simulink model "plant_n"  (R2023a)
settings: Solver=FixedStepAuto  StartTime=0.0  StopTime=200  FixedStep=0.01  RelTol=1e-3
values from neighbouring files (symbols this model uses):
  filter_3 = conv([0.1,1],conv([0.1 1],[0.1 1]))    [main_proj.m]
  filter_x = conv([0.7,1],conv([0.7 1],[0.7 1]))    [main_proj.m]
  kd = 1.117    [main_proj.m]
  ki = 4.47    [main_proj.m]
  kp = 5.366    [main_proj.m]
libraries: neural x772, slpidlib x6
(part 20 of 26)

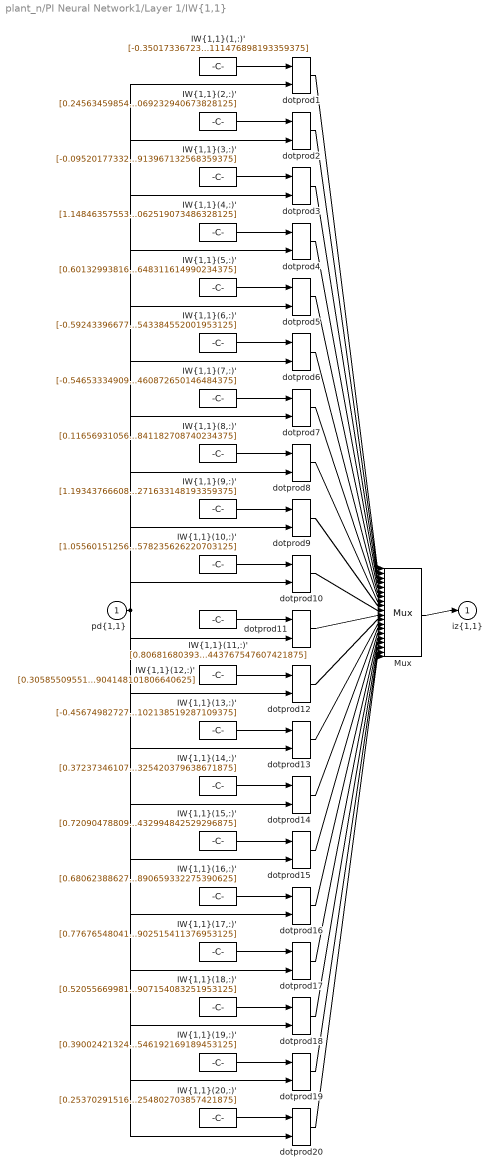
== system plant_n/PI Neural Network1/Layer 1/IW{1,1} ==
  "pd{1,1}" : Inport  PortDimensions=12  SampleTime=0.01
      mask Display: e = 0.06;c1 = [120 230 180]/255;c2 = ([120 230 180]+0)/(256+128);c3 = ([120 230 180]+128)/(256+128);patch([0 1 1 0],[0 0 1 1],c1);patch([0 1 1 1-e 1-e 0+e],[0 0 1 1-e 0+e 0+e],c2);patch([0 0 1 1-e 0+e 0+e],[0 1 1 1-e 1-e 0+e],c3);plot([0 1 1 0 0],[0 0 1 1 0]);
  "IW{1,1}(1,:)'" : Constant  Value=[-0.3501733672305566980043067815131507813930511474609375;0.21065488893706219020174330580630339682102203369140625;-0.210989136698746027054340856921044178307056427001953125;-0.33078704563438676711228936255793087184429168701171875;0.62945158155652103371124894692911766469478607177734375;0.5671066900211059191860840655863285064697265625;0.7803009476457349880007541287341155111789703369140625;-0.168810783126756736027829219892737455666065216064453125;0.980768973519757114587491741986013948917388916015625;-0.84484218705403490989880310735316015779972076416015625;-0.0895432947846148963311208035520394332706928253173828125;-0.9561220185730545662039503440610133111476898193359375]
      mask Display: e = 0.06;c1 = [120 150 230]/255;c2 = ([120 150 230]+0)/383;c3 = ([120 150 230]+128)/383;patch([0 1 1 0],[0 0 1 1],c1);patch([0 1 1 1-e 1-e 0+e],[0 0 1 1-e 0+e 0+e],c2);patch([0 0 1 1-e 0+e 0+e],[0 1 1 1-e 1-e 0+e],c3);plot([0 1 1 0 0],[0 0 1 1 0]);disp('Weights');
  "IW{1,1}(10,:)'" : Constant  Value=[1.05560151256634693339719888172112405300140380859375;0.9332939344408643922434976047952659428119659423828125;-0.277691460157354408355701025357120670378208160400390625;0.7060845075612072196946655822102911770343780517578125;-0.09695879864153743310506428088046959601342678070068359375;-0.2443508749205889341027386763016693294048309326171875;0.367614281091130312706383165277657099068164825439453125;-0.454827087842074317958207529954961501061916351318359375;-0.1513157236805418859315608415272436104714870452880859375;-0.59870946189401774706340120246750302612781524658203125;0.58984455881189068460201951893395744264125823974609375;-0.27134154152465239651093042994034476578235626220703125]
      mask Display: e = 0.06;c1 = [120 150 230]/255;c2 = ([120 150 230]+0)/383;c3 = ([120 150 230]+128)/383;patch([0 1 1 0],[0 0 1 1],c1);patch([0 1 1 1-e 1-e 0+e],[0 0 1 1-e 0+e 0+e],c2);patch([0 0 1 1-e 0+e 0+e],[0 1 1 1-e 1-e 0+e],c3);plot([0 1 1 0 0],[0 0 1 1 0]);disp('Weights');
  "IW{1,1}(11,:)'" : Constant  Value=[0.80681680393463273137655278333113528788089752197265625;0.09439694486195693290397912278422154486179351806640625;-0.77701084247417007144775880078668706119060516357421875;-0.427850899211101032282300593578838743269443511962890625;-0.2232987875497577656691561287516378797590732574462890625;-0.803257944648623212202664944925345480442047119140625;-0.5029394327736536052242399819078855216503143310546875;0.51929065478912439512981791267520748078823089599609375;-0.337093294264546095018175719815189950168132781982421875;-0.834341251775934100720633068704046308994293212890625;0.9091864342576430058073810869245789945125579833984375;-0.89888560861707400562181646819226443767547607421875]
      mask Display: e = 0.06;c1 = [120 150 230]/255;c2 = ([120 150 230]+0)/383;c3 = ([120 150 230]+128)/383;patch([0 1 1 0],[0 0 1 1],c1);patch([0 1 1 1-e 1-e 0+e],[0 0 1 1-e 0+e 0+e],c2);patch([0 0 1 1-e 0+e 0+e],[0 1 1 1-e 1-e 0+e],c3);plot([0 1 1 0 0],[0 0 1 1 0]);disp('Weights');
  "IW{1,1}(12,:)'" : Constant  Value=[0.305855095510365881938952270502340979874134063720703125;0.1233616864154553904864286550946417264640331268310546875;-0.56671614694551519786358539931825362145900726318359375;-0.56492851509072072868633540565497241914272308349609375;0.1722457842120801718710509931042906828224658966064453125;0.63864705288493739399058313210844062268733978271484375;-0.943134606258703822589950505062006413936614990234375;0.80407771540784123143197348326793871819972991943359375;-0.256012471713641887038903632856090553104877471923828125;0.77675127860351655950665872296667657792568206787109375;-0.86701208832907961099323301823460496962070465087890625;0.85618857861038721868141010418185032904148101806640625]
      mask Display: e = 0.06;c1 = [120 150 230]/255;c2 = ([120 150 230]+0)/383;c3 = ([120 150 230]+128)/383;patch([0 1 1 0],[0 0 1 1],c1);patch([0 1 1 1-e 1-e 0+e],[0 0 1 1-e 0+e 0+e],c2);patch([0 0 1 1-e 0+e 0+e],[0 1 1 1-e 1-e 0+e],c3);plot([0 1 1 0 0],[0 0 1 1 0]);disp('Weights');
  "IW{1,1}(13,:)'" : Constant  Value=[-0.456749827277473485764858196489512920379638671875;-0.70461220297198046136344373735482804477214813232421875;-0.209279497403218883722075815967400558292865753173828125;0.41399815885431345829914562273188494145870208740234375;0.89381430939822548165096804950735531747341156005859375;0.84335366269535050331995762462611310184001922607421875;0.0676310309392321451493756967465742491185665130615234375;-0.57820143903720777611709991106181405484676361083984375;0.0861819469902399826199967947104596532881259918212890625;-0.01237860880424513677910969278173070051707327365875244140625;-0.660821274311004902557442619581706821918487548828125;0.35180784796509489975591122856712900102138519287109375]
      mask Display: e = 0.06;c1 = [120 150 230]/255;c2 = ([120 150 230]+0)/383;c3 = ([120 150 230]+128)/383;patch([0 1 1 0],[0 0 1 1],c1);patch([0 1 1 1-e 1-e 0+e],[0 0 1 1-e 0+e 0+e],c2);patch([0 0 1 1-e 0+e 0+e],[0 1 1 1-e 1-e 0+e],c3);plot([0 1 1 0 0],[0 0 1 1 0]);disp('Weights');
  "IW{1,1}(14,:)'" : Constant  Value=[0.372373461077679379638283307940582744777202606201171875;-0.38560447648762530281629778983187861740589141845703125;0.34196789986070263989148543259943835437297821044921875;-0.50526431518178716029154884381568990647792816162109375;-0.167743758165300960172316990792751312255859375;0.84873249279830620395159712643362581729888916015625;-0.94999636271671772380642551070195622742176055908203125;0.860639973471389652104335254989564418792724609375;0.7117112004407477598988407407887279987335205078125;0.97995227919054084253502878709696233272552490234375;-0.4320334908905001380929888910031877458095550537109375;-0.9055841713231955747431811687420122325420379638671875]
      mask Display: e = 0.06;c1 = [120 150 230]/255;c2 = ([120 150 230]+0)/383;c3 = ([120 150 230]+128)/383;patch([0 1 1 0],[0 0 1 1],c1);patch([0 1 1 1-e 1-e 0+e],[0 0 1 1-e 0+e 0+e],c2);patch([0 0 1 1-e 0+e 0+e],[0 1 1 1-e 1-e 0+e],c3);plot([0 1 1 0 0],[0 0 1 1 0]);disp('Weights');
  "IW{1,1}(15,:)'" : Constant  Value=[0.72090478809743185895086980963242240250110626220703125;-0.964711239579766566265561777981929481029510498046875;-0.269719016390192634080591460588038899004459381103515625;-0.245333648835221740380774235745775513350963592529296875;-0.5506486579344376242062253368203528225421905517578125;-0.73357525751399033087096768213086761534214019775390625;0.58313879853820960175170284855994395911693572998046875;0.79142205377866881033099843989475630223751068115234375;0.160230341602728809657918418452027253806591033935546875;0.584078718962899756661499850451946258544921875;0.485155412787328932378017043447471223771572113037109375;0.65783015821145607304742952692322432994842529296875]
      mask Display: e = 0.06;c1 = [120 150 230]/255;c2 = ([120 150 230]+0)/383;c3 = ([120 150 230]+128)/383;patch([0 1 1 0],[0 0 1 1],c1);patch([0 1 1 1-e 1-e 0+e],[0 0 1 1-e 0+e 0+e],c2);patch([0 0 1 1-e 0+e 0+e],[0 1 1 1-e 1-e 0+e],c3);plot([0 1 1 0 0],[0 0 1 1 0]);disp('Weights');
  "IW{1,1}(16,:)'" : Constant  Value=[0.6806238862716977866540446484577842056751251220703125;0.30321005464548689278814208591938950121402740478515625;-0.397392951058915755435663186290184967219829559326171875;-0.372547888856498865539634834931348450481891632080078125;0.1705807666146650081184787950405734591186046600341796875;0.61134879168408728933314932874054647982120513916015625;0.715307662324553117372261112905107438564300537109375;-0.6937658001944537744520857813768088817596435546875;-0.1384741823775422486786368381217471323907375335693359375;-0.5544804190145942168754800150054506957530975341796875;-0.77165132177390471923672521370463073253631591796875;-0.95013052194457225940737998826080001890659332275390625]
      mask Display: e = 0.06;c1 = [120 150 230]/255;c2 = ([120 150 230]+0)/383;c3 = ([120 150 230]+128)/383;patch([0 1 1 0],[0 0 1 1],c1);patch([0 1 1 1-e 1-e 0+e],[0 0 1 1-e 0+e 0+e],c2);patch([0 0 1 1-e 0+e 0+e],[0 1 1 1-e 1-e 0+e],c3);plot([0 1 1 0 0],[0 0 1 1 0]);disp('Weights');
  "IW{1,1}(17,:)'" : Constant  Value=[0.77676548041798110233457919093780219554901123046875;0.59875298284257361114413242830778472125530242919921875;-0.6769123517311761428771887949551455676555633544921875;-0.33193049430556997858587919836281798779964447021484375;-0.818157794952087069617618908523581922054290771484375;-0.488999925412603453356297222853754647076129913330078125;-0.00514354018054317962960197974098264239728450775146484375;0.154838187918311442903274155469262041151523590087890625;-0.1370417754103717411506835333057097159326076507568359375;-0.0833729676382103102039167197290225885808467864990234375;0.2300759161553746212636184509392478503286838531494140625;0.1954796096302804375710593376425094902515411376953125]
      mask Display: e = 0.06;c1 = [120 150 230]/255;c2 = ([120 150 230]+0)/383;c3 = ([120 150 230]+128)/383;patch([0 1 1 0],[0 0 1 1],c1);patch([0 1 1 1-e 1-e 0+e],[0 0 1 1-e 0+e 0+e],c2);patch([0 0 1 1-e 0+e 0+e],[0 1 1 1-e 1-e 0+e],c3);plot([0 1 1 0 0],[0 0 1 1 0]);disp('Weights');
  "IW{1,1}(18,:)'" : Constant  Value=[0.5205566998138924095229640442994423210620880126953125;0.57546124158919287339131187763996422290802001953125;-0.61229287881037508523007772964774630963802337646484375;0.8385272354770882952124111398006789386272430419921875;-0.5968790319572521152480248929350636899471282958984375;-0.6583580586300550319123203735216520726680755615234375;0.77313243054862790248904502732330001890659332275390625;1.03942917397456557893065109965391457080841064453125;-0.4563621264777164565629163917037658393383026123046875;-0.997725917785553750860572108649648725986480712890625;0.32055451180183169856974245703895576298236846923828125;0.3475700277702149509906348612275905907154083251953125]
      mask Display: e = 0.06;c1 = [120 150 230]/255;c2 = ([120 150 230]+0)/383;c3 = ([120 150 230]+128)/383;patch([0 1 1 0],[0 0 1 1],c1);patch([0 1 1 1-e 1-e 0+e],[0 0 1 1-e 0+e 0+e],c2);patch([0 0 1 1-e 0+e 0+e],[0 1 1 1-e 1-e 0+e],c3);plot([0 1 1 0 0],[0 0 1 1 0]);disp('Weights');
  "IW{1,1}(19,:)'" : Constant  Value=[0.39002421324384073386681848205626010894775390625;0.400562910264932792170355924099567346274852752685546875;-0.2375198530981422473384867544154985807836055755615234375;-0.57431896153561778906038171044201590120792388916015625;0.78215669290161271565153811025083996355533599853515625;0.83561444938079942890141182942898012697696685791015625;0.567134150770561173970918389386497437953948974609375;0.47541708112850533662907537291175685822963714599609375;-0.386493398062311310781069551012478768825531005859375;-0.65370461534679957793514404329471290111541748046875;-0.8784701614196148700131061559659428894519805908203125;-0.72780486353654982867311673544463701546192169189453125]
      mask Display: e = 0.06;c1 = [120 150 230]/255;c2 = ([120 150 230]+0)/383;c3 = ([120 150 230]+128)/383;patch([0 1 1 0],[0 0 1 1],c1);patch([0 1 1 1-e 1-e 0+e],[0 0 1 1-e 0+e 0+e],c2);patch([0 0 1 1-e 0+e 0+e],[0 1 1 1-e 1-e 0+e],c3);plot([0 1 1 0 0],[0 0 1 1 0]);disp('Weights');
  "IW{1,1}(2,:)'" : Constant  Value=[0.24563459854675395721557151773595251142978668212890625;-0.426004027323289402584549634411814622581005096435546875;-0.335748503898005423717876283262739889323711395263671875;-0.824260197556788032358099371776916086673736572265625;0.32452062147102489486627518999739550054073333740234375;-0.5366337854891505276810903524165041744709014892578125;0.76409519645451340341679724588175304234027862548828125;0.1301310994903041307058089159909286536276340484619140625;-0.26178114738730895449947411179891787469387054443359375;-0.2031461165731869578099377804392133839428424835205078125;0.498444301046362114870902360053150914609432220458984375;-0.0627893009333209406452880330107291229069232940673828125]
      mask Display: e = 0.06;c1 = [120 150 230]/255;c2 = ([120 150 230]+0)/383;c3 = ([120 150 230]+128)/383;patch([0 1 1 0],[0 0 1 1],c1);patch([0 1 1 1-e 1-e 0+e],[0 0 1 1-e 0+e 0+e],c2);patch([0 0 1 1-e 0+e 0+e],[0 1 1 1-e 1-e 0+e],c3);plot([0 1 1 0 0],[0 0 1 1 0]);disp('Weights');
  "IW{1,1}(20,:)'" : Constant  Value=[0.253702915167598075374399968495708890259265899658203125;-0.5960901430311622561930562369525432586669921875;0.03162143640979653280709271712112240493297576904296875;0.55488413628379540387669521805946715176105499267578125;-0.82497034072777974955670288181863725185394287109375;1.0249513489809498612004290407639928162097930908203125;-0.379953272690083665441562743581016547977924346923828125;-0.50620119900743631990991389102418906986713409423828125;-0.0481707008216175902592937063673161901533603668212890625;0.5965472912594627086235732349450699985027313232421875;0.53990522945679375599326021983870305120944976806640625;-0.33510655264544275677707219074363820254802703857421875]
      mask Display: e = 0.06;c1 = [120 150 230]/255;c2 = ([120 150 230]+0)/383;c3 = ([120 150 230]+128)/383;patch([0 1 1 0],[0 0 1 1],c1);patch([0 1 1 1-e 1-e 0+e],[0 0 1 1-e 0+e 0+e],c2);patch([0 0 1 1-e 0+e 0+e],[0 1 1 1-e 1-e 0+e],c3);plot([0 1 1 0 0],[0 0 1 1 0]);disp('Weights');
  "IW{1,1}(3,:)'" : Constant  Value=[-0.09520177332217207022413418826545239426195621490478515625;0.75088662907703263016401251661591231822967529296875;0.017034568263992501402359636131222941912710666656494140625;-0.047616493164988928088465769405956962145864963531494140625;0.294378828767053402071240952864172868430614471435546875;0.60450574877652918370785073420847766101360321044921875;0.3928392649934309144299504623631946742534637451171875;0.75562967695807536916419167027925141155719757080078125;-0.361625716573649558238656709363567642867565155029296875;-0.055836811852358732288781340002969955094158649444580078125;-0.808722650622968775024901333381421864032745361328125;0.86850949729355020334509163149050436913967132568359375]
      mask Display: e = 0.06;c1 = [120 150 230]/255;c2 = ([120 150 230]+0)/383;c3 = ([120 150 230]+128)/383;patch([0 1 1 0],[0 0 1 1],c1);patch([0 1 1 1-e 1-e 0+e],[0 0 1 1-e 0+e 0+e],c2);patch([0 0 1 1-e 0+e 0+e],[0 1 1 1-e 1-e 0+e],c3);plot([0 1 1 0 0],[0 0 1 1 0]);disp('Weights');
  "IW{1,1}(4,:)'" : Constant  Value=[1.148463575532308045268337082234211266040802001953125;0.1885596221307091202579186983712133951485157012939453125;-0.87683686999453536170534562188549898564815521240234375;0.372542694580555944217081787428469397127628326416015625;-0.9579309956941184367451569414697587490081787109375;0.1281061467383711460765738365807919763028621673583984375;0.8339371150770633622784089311608113348484039306640625;-0.011095559564627939519443344806859386153519153594970703125;-0.47548135283876635792665865665185265243053436279296875;-0.469373337877695695485869009644375182688236236572265625;0.0284250395697532541594565458353827125392854213714599609375;0.81435330892056356777430892179836519062519073486328125]
      mask Display: e = 0.06;c1 = [120 150 230]/255;c2 = ([120 150 230]+0)/383;c3 = ([120 150 230]+128)/383;patch([0 1 1 0],[0 0 1 1],c1);patch([0 1 1 1-e 1-e 0+e],[0 0 1 1-e 0+e 0+e],c2);patch([0 0 1 1-e 0+e 0+e],[0 1 1 1-e 1-e 0+e],c3);plot([0 1 1 0 0],[0 0 1 1 0]);disp('Weights');
  "IW{1,1}(5,:)'" : Constant  Value=[0.60132993816542323894935861972044222056865692138671875;-1.009532261949602105488565939594991505146026611328125;0.4882848557027152924803203859482891857624053955078125;0.1518570495280628929180011255084536969661712646484375;0.00573956743339598153552660875220681191422045230865478515625;0.332422684350621666649061580756097100675106048583984375;0.59046454793114822034993949273484759032726287841796875;0.64171766207403913018225694031571038067340850830078125;0.068993490891669007059050500174635089933872222900390625;1.1388289411276495410874076696927659213542938232421875;-0.72252045473813486520242577171302400529384613037109375;-0.5886223964190671065210835877223871648311614990234375]
      mask Display: e = 0.06;c1 = [120 150 230]/255;c2 = ([120 150 230]+0)/383;c3 = ([120 150 230]+128)/383;patch([0 1 1 0],[0 0 1 1],c1);patch([0 1 1 1-e 1-e 0+e],[0 0 1 1-e 0+e 0+e],c2);patch([0 0 1 1-e 0+e 0+e],[0 1 1 1-e 1-e 0+e],c3);plot([0 1 1 0 0],[0 0 1 1 0]);disp('Weights');
  "IW{1,1}(6,:)'" : Constant  Value=[-0.59243396677047910348079540199250914156436920166015625;-0.09046698029941495355910063835835899226367473602294921875;-0.1323270333664968989584309611018397845327854156494140625;-0.2138507396184003983563570727710612118244171142578125;-0.951443208629644043838879952090792357921600341796875;0.1440957699291008087261189984928932972252368927001953125;-1.031588715944117051748207813943736255168914794921875;-0.619663236082117929726109650800935924053192138671875;0.050268887410226226197806909112841822206974029541015625;0.7071201810445757462986193786491639912128448486328125;0.79706915821870494287537667332799173891544342041015625;0.01299416186979614369623181602264594403095543384552001953125]
      mask Display: e = 0.06;c1 = [120 150 230]/255;c2 = ([120 150 230]+0)/383;c3 = ([120 150 230]+128)/383;patch([0 1 1 0],[0 0 1 1],c1);patch([0 1 1 1-e 1-e 0+e],[0 0 1 1-e 0+e 0+e],c2);patch([0 0 1 1-e 0+e 0+e],[0 1 1 1-e 1-e 0+e],c3);plot([0 1 1 0 0],[0 0 1 1 0]);disp('Weights');
  "IW{1,1}(7,:)'" : Constant  Value=[-0.54653334909987483225535243036574684083461761474609375;-0.82363238945317840400406339540495537221431732177734375;-0.229990176612554109158992332595516927540302276611328125;-0.1575153247271279532970567061056499369442462921142578125;-0.02814796255017969206502215229193097911775112152099609375;0.1620911323758156274976727218017913401126861572265625;0.47864482525470553042623578221537172794342041015625;-0.397873034394290281401396214278065599501132965087890625;0.51155252315615384883784599878708831965923309326171875;0.29100294972542239957391529969754628837108612060546875;-0.797941265801324295381391493720002472400665283203125;0.8305691458852366704235237193643115460872650146484375]
      mask Display: e = 0.06;c1 = [120 150 230]/255;c2 = ([120 150 230]+0)/383;c3 = ([120 150 230]+128)/383;patch([0 1 1 0],[0 0 1 1],c1);patch([0 1 1 1-e 1-e 0+e],[0 0 1 1-e 0+e 0+e],c2);patch([0 0 1 1-e 0+e 0+e],[0 1 1 1-e 1-e 0+e],c3);plot([0 1 1 0 0],[0 0 1 1 0]);disp('Weights');
  "IW{1,1}(8,:)'" : Constant  Value=[0.1165693105668253182205518214686890132725238800048828125;0.420668433343472536467544387051020748913288116455078125;-0.2082148171276476389390808208190719597041606903076171875;0.71054384066538400777091055715573020279407501220703125;-0.9019385684760774513080150427413173019886016845703125;0.71615432960772285042594376136548817157745361328125;0.497350539421919035643071538288495503365993499755859375;-0.33943619664990964945872065072762779891490936279296875;0.92558836246940578984521152960951440036296844482421875;0.0110971454482443922240353373354082577861845493316650390625;0.59181877682224792724952067146659828722476959228515625;-0.75010903121931116199760936069651506841182708740234375]
      mask Display: e = 0.06;c1 = [120 150 230]/255;c2 = ([120 150 230]+0)/383;c3 = ([120 150 230]+128)/383;patch([0 1 1 0],[0 0 1 1],c1);patch([0 1 1 1-e 1-e 0+e],[0 0 1 1-e 0+e 0+e],c2);patch([0 0 1 1-e 0+e 0+e],[0 1 1 1-e 1-e 0+e],c3);plot([0 1 1 0 0],[0 0 1 1 0]);disp('Weights');
  "IW{1,1}(9,:)'" : Constant  Value=[1.193437666082116432875181999406777322292327880859375;0.2986136361520810300618222754565067589282989501953125;0.70220141834500393596130152218393050134181976318359375;0.40445185365829694479344880164717324078083038330078125;0.190528694302082801659281585671124048531055450439453125;0.3966708645648961972796087138704024255275726318359375;0.862038699213499182150144406477920711040496826171875;-0.615984327445402879419589226017706096172332763671875;-0.59179765138318030093245170064619742333889007568359375;-0.49671077030633858928609924987540580332279205322265625;0.78599527396450585836618074608850292861461639404296875;-0.99505520787260903770032882675877772271633148193359375]
      mask Display: e = 0.06;c1 = [120 150 230]/255;c2 = ([120 150 230]+0)/383;c3 = ([120 150 230]+128)/383;patch([0 1 1 0],[0 0 1 1],c1);patch([0 1 1 1-e 1-e 0+e],[0 0 1 1-e 0+e 0+e],c2);patch([0 0 1 1-e 0+e 0+e],[0 1 1 1-e 1-e 0+e],c3);plot([0 1 1 0 0],[0 0 1 1 0]);disp('Weights');
  Mux : Mux  Inputs=20
      mask Display: e = 0.06;c1 = [120 150 230]/255;c2 = ([120 150 230]+0)/383;c3 = ([120 150 230]+128)/383;patch([0 1 1 0],[0 0 1 1],c1);patch([0 1 1 1-e 1-e 0+e],[0 0 1 1-e 0+e 0+e],c2);patch([0 0 1 1-e 0+e 0+e],[0 1 1 1-e 1-e 0+e],c3);plot([0 1 1 0 0],[0 0 1 1 0]);disp('Mux');
  dotprod{1..20} (20 alike) : neural/Weight Functions/dotprod
  "iz{1,1}" : Outport
      mask Display: e = 0.06;c1 = [120 230 180]/255;c2 = ([120 230 180]+0)/(256+128);c3 = ([120 230 180]+128)/(256+128);patch([0 1 1 0],[0 0 1 1],c1);patch([0 1 1 1-e 1-e 0+e],[0 0 1 1-e 0+e 0+e],c2);patch([0 0 1 1-e 0+e 0+e],[0 1 1 1-e 1-e 0+e],c3);plot([0 1 1 0 0],[0 0 1 1 0]);
  wires:
  Mux/1 -> "iz{1,1}"/1
  dotprod20/1 -> Mux/20
  "IW{1,1}(20,:)'"/1 -> dotprod20/1
  dotprod19/1 -> Mux/19
  "IW{1,1}(19,:)'"/1 -> dotprod19/1
  dotprod18/1 -> Mux/18
  "IW{1,1}(18,:)'"/1 -> dotprod18/1
  dotprod17/1 -> Mux/17
  "IW{1,1}(17,:)'"/1 -> dotprod17/1
  dotprod16/1 -> Mux/16
  "IW{1,1}(16,:)'"/1 -> dotprod16/1
  dotprod15/1 -> Mux/15
  "IW{1,1}(15,:)'"/1 -> dotprod15/1
  dotprod14/1 -> Mux/14
  "IW{1,1}(14,:)'"/1 -> dotprod14/1
  dotprod13/1 -> Mux/13
  "IW{1,1}(13,:)'"/1 -> dotprod13/1
  dotprod12/1 -> Mux/12
  "IW{1,1}(12,:)'"/1 -> dotprod12/1
  dotprod11/1 -> Mux/11
  "IW{1,1}(11,:)'"/1 -> dotprod11/1
  dotprod10/1 -> Mux/10
  "IW{1,1}(10,:)'"/1 -> dotprod10/1
  dotprod9/1 -> Mux/9
  "IW{1,1}(9,:)'"/1 -> dotprod9/1
  dotprod8/1 -> Mux/8
  "IW{1,1}(8,:)'"/1 -> dotprod8/1
  dotprod7/1 -> Mux/7
  "IW{1,1}(7,:)'"/1 -> dotprod7/1
  dotprod6/1 -> Mux/6
  "IW{1,1}(6,:)'"/1 -> dotprod6/1
  dotprod5/1 -> Mux/5
  "IW{1,1}(5,:)'"/1 -> dotprod5/1
  dotprod4/1 -> Mux/4
  "IW{1,1}(4,:)'"/1 -> dotprod4/1
  dotprod3/1 -> Mux/3
  "IW{1,1}(3,:)'"/1 -> dotprod3/1
  dotprod2/1 -> Mux/2
  "IW{1,1}(2,:)'"/1 -> dotprod2/1
  dotprod1/1 -> Mux/1
  "pd{1,1}"/1 -> dotprod20/2, dotprod19/2, dotprod18/2, dotprod17/2, dotprod16/2, dotprod15/2, dotprod14/2, dotprod13/2, dotprod12/2, dotprod11/2, dotprod10/2, dotprod9/2, dotprod8/2, dotprod7/2, dotprod6/2, dotprod5/2, dotprod4/2, dotprod3/2, dotprod2/2, dotprod1/2
  "IW{1,1}(1,:)'"/1 -> dotprod1/1

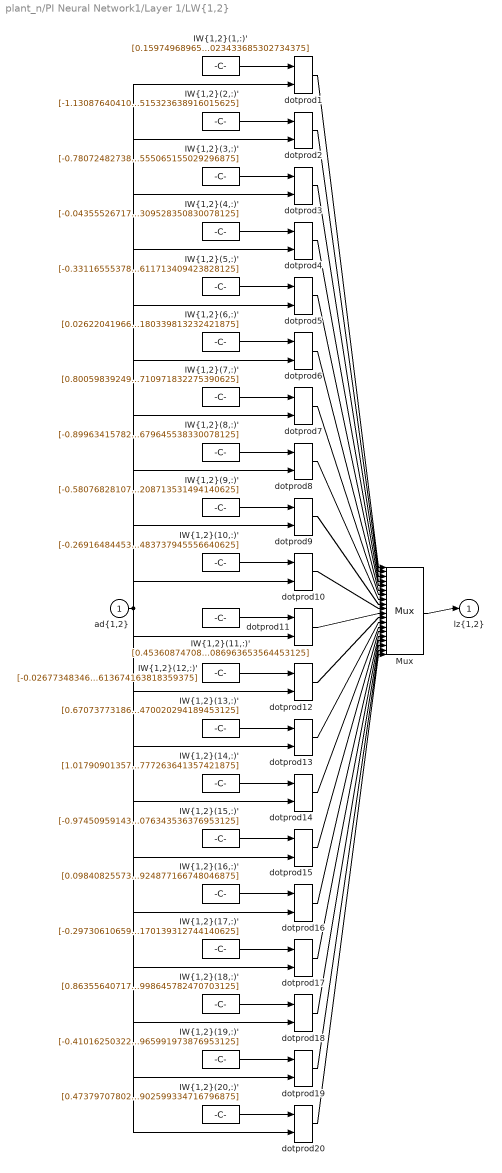
== system plant_n/PI Neural Network1/Layer 1/LW{1,2} ==
  "ad{1,2}" : Inport  PortDimensions=12  SampleTime=0.01
      mask Display: e = 0.06;c1 = [120 230 180]/255;c2 = ([120 230 180]+0)/(256+128);c3 = ([120 230 180]+128)/(256+128);patch([0 1 1 0],[0 0 1 1],c1);patch([0 1 1 1-e 1-e 0+e],[0 0 1 1-e 0+e 0+e],c2);patch([0 0 1 1-e 0+e 0+e],[0 1 1 1-e 1-e 0+e],c3);plot([0 1 1 0 0],[0 0 1 1 0]);
  "IW{1,2}(1,:)'" : Constant  Value=[0.1597496896582787095919542252886458300054073333740234375;-0.1444840271877911863640520095941610634326934814453125;0.73753415860299231798791197434184141457080841064453125;0.06361365398029507345345479052411974407732486724853515625;0.62317568056404459841957077514962293207645416259765625;-0.91143253493693998645852616391493938863277435302734375;0.82264716058652698205122533181565813720226287841796875;-0.64712311433395675042135053445235826075077056884765625;0.50318712354767669570065891093690879642963409423828125;-0.3970278810703471439325085157179273664951324462890625;0.563337937916049913411598026868887245655059814453125;0.9895208016848666687792501761578023433685302734375]
      mask Display: e = 0.06;c1 = [120 150 230]/255;c2 = ([120 150 230]+0)/383;c3 = ([120 150 230]+128)/383;patch([0 1 1 0],[0 0 1 1],c1);patch([0 1 1 1-e 1-e 0+e],[0 0 1 1-e 0+e 0+e],c2);patch([0 0 1 1-e 0+e 0+e],[0 1 1 1-e 1-e 0+e],c3);plot([0 1 1 0 0],[0 0 1 1 0]);disp('weights');
  "IW{1,2}(10,:)'" : Constant  Value=[-0.269164844537187419870605253890971653163433074951171875;0.08250398841647203773685959049544180743396282196044921875;-0.06730380368054700301883030988392420113086700439453125;0.18151356321064238130702506168745458126068115234375;0.492956593845259527508773089721216820180416107177734375;-0.67956812408399558389504591104923747479915618896484375;-0.58673899169878895865082313321181572973728179931640625;-0.76305811680621804526936102774925529956817626953125;-0.11112826248269895568210330338843050412833690643310546875;0.54558672479518122155894843672285787761211395263671875;-0.292202165862956053654642118999618105590343475341796875;-0.407571827996035696006771331667550839483737945556640625]
      mask Display: e = 0.06;c1 = [120 150 230]/255;c2 = ([120 150 230]+0)/383;c3 = ([120 150 230]+128)/383;patch([0 1 1 0],[0 0 1 1],c1);patch([0 1 1 1-e 1-e 0+e],[0 0 1 1-e 0+e 0+e],c2);patch([0 0 1 1-e 0+e 0+e],[0 1 1 1-e 1-e 0+e],c3);plot([0 1 1 0 0],[0 0 1 1 0]);disp('weights');
  "IW{1,2}(11,:)'" : Constant  Value=[0.45360874708614506989334813624736852943897247314453125;-0.68976883330267757532539008025196380913257598876953125;0.2855567985304079403618970900424756109714508056640625;0.005183082715861159726900009303562910645268857479095458984375;0.840020822301740022197691359906457364559173583984375;0.62254590404124809932540074441931210458278656005859375;0.335603676854137555896073763506137765944004058837890625;0.134497811711054016114985643071122467517852783203125;-1.0108627689599842813805707919527776539325714111328125;0.269695280599674791499609227685141377151012420654296875;0.56561635199126047979234499507583677768707275390625;0.265878412383234508098439619061537086963653564453125]
      mask Display: e = 0.06;c1 = [120 150 230]/255;c2 = ([120 150 230]+0)/383;c3 = ([120 150 230]+128)/383;patch([0 1 1 0],[0 0 1 1],c1);patch([0 1 1 1-e 1-e 0+e],[0 0 1 1-e 0+e 0+e],c2);patch([0 0 1 1-e 0+e 0+e],[0 1 1 1-e 1-e 0+e],c3);plot([0 1 1 0 0],[0 0 1 1 0]);disp('weights');
  "IW{1,2}(12,:)'" : Constant  Value=[-0.0267734834665425587563181153427649405784904956817626953125;-0.997611503952075207024563496815972030162811279296875;-0.362034515980711069094155618586228229105472564697265625;0.90652221298317614550654752747504971921443939208984375;0.65559596385809515428633176270523108541965484619140625;-0.216720919999064454142256863633519969880580902099609375;0.335051010770904877933418219981831498444080352783203125;0.03183049231912309096070856639926205389201641082763671875;-0.5947708157250379823466346351779066026210784912109375;-0.4793344294483998790923351407400332391262054443359375;0.6939218403823261827056967376847751438617706298828125;-0.44934155038149581340434224330238066613674163818359375]
      mask Display: e = 0.06;c1 = [120 150 230]/255;c2 = ([120 150 230]+0)/383;c3 = ([120 150 230]+128)/383;patch([0 1 1 0],[0 0 1 1],c1);patch([0 1 1 1-e 1-e 0+e],[0 0 1 1-e 0+e 0+e],c2);patch([0 0 1 1-e 0+e 0+e],[0 1 1 1-e 1-e 0+e],c3);plot([0 1 1 0 0],[0 0 1 1 0]);disp('weights');
  "IW{1,2}(13,:)'" : Constant  Value=[0.6707377318614982097955135031952522695064544677734375;-0.134645366751897033186224916789797134697437286376953125;0.912407170276967605104800895787775516510009765625;-0.1232787635037957130190733323615859262645244598388671875;-0.1851363096097623228697415243004797957837581634521484375;-0.01480114129923651260234418458594518597237765789031982421875;-0.13605405074537235687870406763977371156215667724609375;-0.96698033264475491410649965473567135632038116455078125;0.6052550060537187359699373701005242764949798583984375;0.453785075586198349828492837332305498421192169189453125;-0.85731674936075152881898020496009849011898040771484375;0.493562363027554074079716883716173470020294189453125]
      mask Display: e = 0.06;c1 = [120 150 230]/255;c2 = ([120 150 230]+0)/383;c3 = ([120 150 230]+128)/383;patch([0 1 1 0],[0 0 1 1],c1);patch([0 1 1 1-e 1-e 0+e],[0 0 1 1-e 0+e 0+e],c2);patch([0 0 1 1-e 0+e 0+e],[0 1 1 1-e 1-e 0+e],c3);plot([0 1 1 0 0],[0 0 1 1 0]);disp('weights');
  "IW{1,2}(14,:)'" : Constant  Value=[1.0179090135748649625924144856981001794338226318359375;-0.311823646676756716100697985893930308520793914794921875;-0.11392542718795158063205263943018508143723011016845703125;0.278749101645987151787409175085485912859439849853515625;-0.97050516771337524968288335003308020532131195068359375;0.41365938110056965637539860836113803088665008544921875;-0.440981425418894179557582901907153427600860595703125;0.9670687980660819249578707967884838581085205078125;0.78103856202226074056937932255095802247524261474609375;-0.922158805748736210006200053612701594829559326171875;-0.77781997748178033358357197357690893113613128662109375;-0.32243917896875096129605253736372105777263641357421875]
      mask Display: e = 0.06;c1 = [120 150 230]/255;c2 = ([120 150 230]+0)/383;c3 = ([120 150 230]+128)/383;patch([0 1 1 0],[0 0 1 1],c1);patch([0 1 1 1-e 1-e 0+e],[0 0 1 1-e 0+e 0+e],c2);patch([0 0 1 1-e 0+e 0+e],[0 1 1 1-e 1-e 0+e],c3);plot([0 1 1 0 0],[0 0 1 1 0]);disp('weights');
  "IW{1,2}(15,:)'" : Constant  Value=[-0.97450959143104742832264264507102780044078826904296875;-0.70555592259081445494217632585787214338779449462890625;0.53817891822856911421268932826933450996875762939453125;0.906715088050710438238866117899306118488311767578125;0.33585549786678059458466805153875611722469329833984375;0.18409855322441626146456883361679501831531524658203125;0.5030938488890759341387592940009199082851409912109375;0.8540454421107870341955958792823366820812225341796875;-0.72485200139557026677294970795628614723682403564453125;0.1499766208486572327540642390886205248534679412841796875;0.70730378301279994701644682209007441997528076171875;-0.9700243958484240369699591610697098076343536376953125]
      mask Display: e = 0.06;c1 = [120 150 230]/255;c2 = ([120 150 230]+0)/383;c3 = ([120 150 230]+128)/383;patch([0 1 1 0],[0 0 1 1],c1);patch([0 1 1 1-e 1-e 0+e],[0 0 1 1-e 0+e 0+e],c2);patch([0 0 1 1-e 0+e 0+e],[0 1 1 1-e 1-e 0+e],c3);plot([0 1 1 0 0],[0 0 1 1 0]);disp('weights');
  "IW{1,2}(16,:)'" : Constant  Value=[0.0984082557360545784330696506003732793033123016357421875;0.07112267167603082695936933532721013762056827545166015625;-0.985478155285105739125128820887766778469085693359375;0.54955708641358480548433362855575978755950927734375;-0.058646579512673192857707960001789615489542484283447265625;0.84360331112003195119797283041407354176044464111328125;-1.011930197528680519525323688867501914501190185546875;0.31158917370025063231508966055116616189479827880859375;0.29007392299496459475705023578484542667865753173828125;0.66946726270320822127501969589502550661563873291015625;-0.8880057897408988321075185012887232005596160888671875;0.04844420058327518485707940953943761996924877166748046875]
      mask Display: e = 0.06;c1 = [120 150 230]/255;c2 = ([120 150 230]+0)/383;c3 = ([120 150 230]+128)/383;patch([0 1 1 0],[0 0 1 1],c1);patch([0 1 1 1-e 1-e 0+e],[0 0 1 1-e 0+e 0+e],c2);patch([0 0 1 1-e 0+e 0+e],[0 1 1 1-e 1-e 0+e],c3);plot([0 1 1 0 0],[0 0 1 1 0]);disp('weights');
  "IW{1,2}(17,:)'" : Constant  Value=[-0.297306106595756902688520995070575736463069915771484375;-0.21632233802204436923233288325718604028224945068359375;-0.53225032917665815457297640023170970380306243896484375;-0.56227523170238213889859935079584829509258270263671875;0.2078344373792150034940817704409710131585597991943359375;-0.037441594107742288966012011997008812613785266876220703125;-0.37302281414067139930779148926376365125179290771484375;0.65132124900377952325669639321858994662761688232421875;0.1704244181983730899165863093003281392157077789306640625;0.308960410486835812537975698433001525700092315673828125;0.0835370024553648005127826081661623902618885040283203125;0.051591211895042544954836927217911579646170139312744140625]
      mask Display: e = 0.06;c1 = [120 150 230]/255;c2 = ([120 150 230]+0)/383;c3 = ([120 150 230]+128)/383;patch([0 1 1 0],[0 0 1 1],c1);patch([0 1 1 1-e 1-e 0+e],[0 0 1 1-e 0+e 0+e],c2);patch([0 0 1 1-e 0+e 0+e],[0 1 1 1-e 1-e 0+e],c3);plot([0 1 1 0 0],[0 0 1 1 0]);disp('weights');
  "IW{1,2}(18,:)'" : Constant  Value=[0.8635564071762795723685712800943292677402496337890625;0.54709238615447952636117179281427524983882904052734375;-0.58928508205499241512370645068585872650146484375;0.92405098488025549929858470932231284677982330322265625;-0.4763102801653917861557374635594896972179412841796875;0.474769096583644134579316187227959744632244110107421875;0.8262005161740140213311178740696050226688385009765625;-0.575996433186215739397084689699113368988037109375;0.195217786411381710731660632518469356000423431396484375;0.453235612513086250086047357399365864694118499755859375;0.411327131043432103751911199651658535003662109375;0.662000841015040197845564762246794998645782470703125]
      mask Display: e = 0.06;c1 = [120 150 230]/255;c2 = ([120 150 230]+0)/383;c3 = ([120 150 230]+128)/383;patch([0 1 1 0],[0 0 1 1],c1);patch([0 1 1 1-e 1-e 0+e],[0 0 1 1-e 0+e 0+e],c2);patch([0 0 1 1-e 0+e 0+e],[0 1 1 1-e 1-e 0+e],c3);plot([0 1 1 0 0],[0 0 1 1 0]);disp('weights');
  "IW{1,2}(19,:)'" : Constant  Value=[-0.410162503226807750866811375090037472546100616455078125;-0.6654357843721270260317623979062773287296295166015625;-0.82249364003484959351197858268278650939464569091796875;0.226965109049404423213758263955242000520229339599609375;0.472471148748886349277853469175170175731182098388671875;0.164156282323860980287832944668480195105075836181640625;-0.82787726071609346600865819709724746644496917724609375;-0.98246189769805181146722361518186517059803009033203125;0.329906582291327132860914161938126198947429656982421875;-0.93270309342479984504592493976815603673458099365234375;0.50482058587788258829931464788387529551982879638671875;0.1720564690664943274800435801807907409965991973876953125]
      mask Display: e = 0.06;c1 = [120 150 230]/255;c2 = ([120 150 230]+0)/383;c3 = ([120 150 230]+128)/383;patch([0 1 1 0],[0 0 1 1],c1);patch([0 1 1 1-e 1-e 0+e],[0 0 1 1-e 0+e 0+e],c2);patch([0 0 1 1-e 0+e 0+e],[0 1 1 1-e 1-e 0+e],c3);plot([0 1 1 0 0],[0 0 1 1 0]);disp('weights');
  "IW{1,2}(2,:)'" : Constant  Value=[-1.1308764041020820112493083797744475305080413818359375;0.4352367776573016211472122449777089059352874755859375;0.19763974958758423472460208358825184404850006103515625;0.37392719380558603337050271875341422855854034423828125;-0.34832754597812665142697596820653416216373443603515625;0.5962392023114333472477710529346950352191925048828125;0.46700266255980793506097370482166297733783721923828125;-0.64710565784694928925802059893612749874591827392578125;-0.55198631395046771075385549920611083507537841796875;0.2418627868763673360863464267822564579546451568603515625;0.2829788765706273689914951319224201142787933349609375;-0.81470662630979318041823944440693594515323638916015625]
      mask Display: e = 0.06;c1 = [120 150 230]/255;c2 = ([120 150 230]+0)/383;c3 = ([120 150 230]+128)/383;patch([0 1 1 0],[0 0 1 1],c1);patch([0 1 1 1-e 1-e 0+e],[0 0 1 1-e 0+e 0+e],c2);patch([0 0 1 1-e 0+e 0+e],[0 1 1 1-e 1-e 0+e],c3);plot([0 1 1 0 0],[0 0 1 1 0]);disp('weights');
  "IW{1,2}(20,:)'" : Constant  Value=[0.47379707802890880241619697699206881225109100341796875;0.1301103974051512068843550196106662042438983917236328125;-0.8127442842886123397505571119836531579494476318359375;0.09998164948722021438953788674552924931049346923828125;0.09739117899433587244306664842952159233391284942626953125;-0.92496936337026713914610809297300875186920166015625;-0.68811718715722680617119522139546461403369903564453125;-0.76487647030329952713145758025348186492919921875;0.5909197241367747377438490730128251016139984130859375;-0.95878898100849685448565651313401758670806884765625;0.5225015361384677259337649957160465419292449951171875;-0.472802954028870903169234907181817106902599334716796875]
      mask Display: e = 0.06;c1 = [120 150 230]/255;c2 = ([120 150 230]+0)/383;c3 = ([120 150 230]+128)/383;patch([0 1 1 0],[0 0 1 1],c1);patch([0 1 1 1-e 1-e 0+e],[0 0 1 1-e 0+e 0+e],c2);patch([0 0 1 1-e 0+e 0+e],[0 1 1 1-e 1-e 0+e],c3);plot([0 1 1 0 0],[0 0 1 1 0]);disp('weights');
  "IW{1,2}(3,:)'" : Constant  Value=[-0.7807248273876170596707879667519591748714447021484375;0.57171880202164260253994143567979335784912109375;0.3487767847999172499129372226889245212078094482421875;-0.73706437945092917463085768758901394903659820556640625;0.686119903240882234030095787602476775646209716796875;0.0901658856658094365332800634860177524387836456298828125;-0.194331543305954645983746331694419495761394500732421875;0.84613406987719519403157164560980163514614105224609375;-0.59594310004539308156523702564300037920475006103515625;0.355065382604327572924063360915170051157474517822265625;-0.01684656415909820126319829114436288364231586456298828125;-0.6371255963756237150619199383072555065155029296875]
      mask Display: e = 0.06;c1 = [120 150 230]/255;c2 = ([120 150 230]+0)/383;c3 = ([120 150 230]+128)/383;patch([0 1 1 0],[0 0 1 1],c1);patch([0 1 1 1-e 1-e 0+e],[0 0 1 1-e 0+e 0+e],c2);patch([0 0 1 1-e 0+e 0+e],[0 1 1 1-e 1-e 0+e],c3);plot([0 1 1 0 0],[0 0 1 1 0]);disp('weights');
  "IW{1,2}(4,:)'" : Constant  Value=[-0.043555267178964705843124960438217385672032833099365234375;0.024928405157204132358561565752097521908581256866455078125;-0.62391235978996240074678780729300342500209808349609375;0.186975524034526385808163695401162840425968170166015625;-0.0096840179012096759547656432687290362082421779632568359375;1.06241655228377585018506579217500984668731689453125;-0.040483711109536059391533768803128623403608798980712890625;0.0417583151937868934933106856988160870969295501708984375;0.442015278476706630073067572084255516529083251953125;0.97051689697679355273152168592787347733974456787109375;0.426615566182979411014031256854650564491748809814453125;-0.5042305660825683322201484770630486309528350830078125]
      mask Display: e = 0.06;c1 = [120 150 230]/255;c2 = ([120 150 230]+0)/383;c3 = ([120 150 230]+128)/383;patch([0 1 1 0],[0 0 1 1],c1);patch([0 1 1 1-e 1-e 0+e],[0 0 1 1-e 0+e 0+e],c2);patch([0 0 1 1-e 0+e 0+e],[0 1 1 1-e 1-e 0+e],c3);plot([0 1 1 0 0],[0 0 1 1 0]);disp('weights');
  "IW{1,2}(5,:)'" : Constant  Value=[-0.33116555378718270929994105244986712932586669921875;-0.60356454531992309586740930171799845993518829345703125;0.334319852599775535484383226503268815577030181884765625;0.257862476522496775199755347784957848489284515380859375;-0.3757003553553504016093711470603011548519134521484375;-0.650612330043602415940995342680253088474273681640625;0.236295801735354304984326745397993363440036773681640625;0.5715148437557104887929426695336587727069854736328125;-0.332157276480056662393280930700711905956268310546875;0.54245117568653078432561187582905404269695281982421875;-0.7800832714863681349726221014861948788166046142578125;-0.65833779525094471285484587497194297611713409423828125]
      mask Display: e = 0.06;c1 = [120 150 230]/255;c2 = ([120 150 230]+0)/383;c3 = ([120 150 230]+128)/383;patch([0 1 1 0],[0 0 1 1],c1);patch([0 1 1 1-e 1-e 0+e],[0 0 1 1-e 0+e 0+e],c2);patch([0 0 1 1-e 0+e 0+e],[0 1 1 1-e 1-e 0+e],c3);plot([0 1 1 0 0],[0 0 1 1 0]);disp('weights');
  "IW{1,2}(6,:)'" : Constant  Value=[0.02622041966575770766123554267323925159871578216552734375;0.047417367958261201488223690603263094089925289154052734375;-0.2115522807242431191365739095999742858111858367919921875;-0.58702614509412864851611857375246472656726837158203125;-0.73659271465842068860041536026983521878719329833984375;0.1964128051472327218807123472288367338478565216064453125;0.5078985531408719555912512078066356480121612548828125;0.288868466843485272033120736523414961993694305419921875;-0.1022073318490643867306744141387753188610076904296875;-0.91034191594624525034618045538081787526607513427734375;-0.8020554644716562098238910039071924984455108642578125;-0.5733272113679230841398748452775180339813232421875]
      mask Display: e = 0.06;c1 = [120 150 230]/255;c2 = ([120 150 230]+0)/383;c3 = ([120 150 230]+128)/383;patch([0 1 1 0],[0 0 1 1],c1);patch([0 1 1 1-e 1-e 0+e],[0 0 1 1-e 0+e 0+e],c2);patch([0 0 1 1-e 0+e 0+e],[0 1 1 1-e 1-e 0+e],c3);plot([0 1 1 0 0],[0 0 1 1 0]);disp('weights');
  "IW{1,2}(7,:)'" : Constant  Value=[0.80059839249225728252667977358214557170867919921875;0.61551371837840207490444299764931201934814453125;-0.299102871071125375745936025850824080407619476318359375;0.49841253509289551448802058075671084225177764892578125;-0.047892367685029059443113652605461538769304752349853515625;-0.59045235443250387863400874266517348587512969970703125;0.62915309379828132652079375475295819342136383056640625;-0.5383114485199607113230513277812860906124114990234375;0.56091125966683763603981560663669370114803314208984375;0.27595457650631616264291778861661441624164581298828125;0.102430983611131953825434948157635517418384552001953125;0.5160422928146284338168925387435592710971832275390625]
      mask Display: e = 0.06;c1 = [120 150 230]/255;c2 = ([120 150 230]+0)/383;c3 = ([120 150 230]+128)/383;patch([0 1 1 0],[0 0 1 1],c1);patch([0 1 1 1-e 1-e 0+e],[0 0 1 1-e 0+e 0+e],c2);patch([0 0 1 1-e 0+e 0+e],[0 1 1 1-e 1-e 0+e],c3);plot([0 1 1 0 0],[0 0 1 1 0]);disp('weights');
  "IW{1,2}(8,:)'" : Constant  Value=[-0.89963415782252287300480020348913967609405517578125;0.07984383712378502473416830298447166569530963897705078125;0.0202391564880668971271315825788406073115766048431396484375;-0.023096881144017589182482197429635562002658843994140625;0.163403613051667451205872794162132777273654937744140625;-0.2714535968926077291740739383385516703128814697265625;0.71100931097378661238650465747923590242862701416015625;-0.61534555507792443318493269543978385627269744873046875;0.1035889640253845056516723843742511235177516937255859375;-0.518637213479620218237187145859934389591217041015625;0.8162964668221268649261901373392902314662933349609375;0.67316807580310034087034409822081215679645538330078125]
      mask Display: e = 0.06;c1 = [120 150 230]/255;c2 = ([120 150 230]+0)/383;c3 = ([120 150 230]+128)/383;patch([0 1 1 0],[0 0 1 1],c1);patch([0 1 1 1-e 1-e 0+e],[0 0 1 1-e 0+e 0+e],c2);patch([0 0 1 1-e 0+e 0+e],[0 1 1 1-e 1-e 0+e],c3);plot([0 1 1 0 0],[0 0 1 1 0]);disp('weights');
  "IW{1,2}(9,:)'" : Constant  Value=[-0.5807682810780072646394955881987698376178741455078125;0.95954816916592433617694268832565285265445709228515625;-0.6725202527095250903954593013622798025608062744140625;0.51393008666567652209522520934115163981914520263671875;-0.330582438665093292229357757605612277984619140625;0.657577640470357049906624524737708270549774169921875;0.11730490791532889593984378961977199651300907135009765625;-0.33086070298579439707964411354623734951019287109375;-0.461414614923287447201261102236458100378513336181640625;-0.6960131687436332814655770562239922583103179931640625;1.0138053890387919153681650641374289989471435546875;-0.56592213481830599963728900547721423208713531494140625]
      mask Display: e = 0.06;c1 = [120 150 230]/255;c2 = ([120 150 230]+0)/383;c3 = ([120 150 230]+128)/383;patch([0 1 1 0],[0 0 1 1],c1);patch([0 1 1 1-e 1-e 0+e],[0 0 1 1-e 0+e 0+e],c2);patch([0 0 1 1-e 0+e 0+e],[0 1 1 1-e 1-e 0+e],c3);plot([0 1 1 0 0],[0 0 1 1 0]);disp('weights');
  Mux : Mux  Inputs=20
      mask Display: e = 0.06;c1 = [120 150 230]/255;c2 = ([120 150 230]+0)/383;c3 = ([120 150 230]+128)/383;patch([0 1 1 0],[0 0 1 1],c1);patch([0 1 1 1-e 1-e 0+e],[0 0 1 1-e 0+e 0+e],c2);patch([0 0 1 1-e 0+e 0+e],[0 1 1 1-e 1-e 0+e],c3);plot([0 1 1 0 0],[0 0 1 1 0]);disp('Mux');
  dotprod{1..20} (20 alike) : neural/Weight Functions/dotprod
  "lz{1,2}" : Outport
      mask Display: e = 0.06;c1 = [120 230 180]/255;c2 = ([120 230 180]+0)/(256+128);c3 = ([120 230 180]+128)/(256+128);patch([0 1 1 0],[0 0 1 1],c1);patch([0 1 1 1-e 1-e 0+e],[0 0 1 1-e 0+e 0+e],c2);patch([0 0 1 1-e 0+e 0+e],[0 1 1 1-e 1-e 0+e],c3);plot([0 1 1 0 0],[0 0 1 1 0]);
  wires:
  Mux/1 -> "lz{1,2}"/1
  dotprod20/1 -> Mux/20
  "IW{1,2}(20,:)'"/1 -> dotprod20/1
  dotprod19/1 -> Mux/19
  "IW{1,2}(19,:)'"/1 -> dotprod19/1
  dotprod18/1 -> Mux/18
  "IW{1,2}(18,:)'"/1 -> dotprod18/1
  dotprod17/1 -> Mux/17
  "IW{1,2}(17,:)'"/1 -> dotprod17/1
  dotprod16/1 -> Mux/16
  "IW{1,2}(16,:)'"/1 -> dotprod16/1
  dotprod15/1 -> Mux/15
  "IW{1,2}(15,:)'"/1 -> dotprod15/1
  dotprod14/1 -> Mux/14
  "IW{1,2}(14,:)'"/1 -> dotprod14/1
  dotprod13/1 -> Mux/13
  "IW{1,2}(13,:)'"/1 -> dotprod13/1
  dotprod12/1 -> Mux/12
  "IW{1,2}(12,:)'"/1 -> dotprod12/1
  dotprod11/1 -> Mux/11
  "IW{1,2}(11,:)'"/1 -> dotprod11/1
  dotprod10/1 -> Mux/10
  "IW{1,2}(10,:)'"/1 -> dotprod10/1
  dotprod9/1 -> Mux/9
  "IW{1,2}(9,:)'"/1 -> dotprod9/1
  dotprod8/1 -> Mux/8
  "IW{1,2}(8,:)'"/1 -> dotprod8/1
  dotprod7/1 -> Mux/7
  "IW{1,2}(7,:)'"/1 -> dotprod7/1
  dotprod6/1 -> Mux/6
  "IW{1,2}(6,:)'"/1 -> dotprod6/1
  dotprod5/1 -> Mux/5
  "IW{1,2}(5,:)'"/1 -> dotprod5/1
  dotprod4/1 -> Mux/4
  "IW{1,2}(4,:)'"/1 -> dotprod4/1
  dotprod3/1 -> Mux/3
  "IW{1,2}(3,:)'"/1 -> dotprod3/1
  dotprod2/1 -> Mux/2
  "IW{1,2}(2,:)'"/1 -> dotprod2/1
  dotprod1/1 -> Mux/1
  "ad{1,2}"/1 -> dotprod20/2, dotprod19/2, dotprod18/2, dotprod17/2, dotprod16/2, dotprod15/2, dotprod14/2, dotprod13/2, dotprod12/2, dotprod11/2, dotprod10/2, dotprod9/2, dotprod8/2, dotprod7/2, dotprod6/2, dotprod5/2, dotprod4/2, dotprod3/2, dotprod2/2, dotprod1/2
  "IW{1,2}(1,:)'"/1 -> dotprod1/1

== system plant_n/PI Neural Network1/Layer 2/Delays 1 ==
  "p{2}" : Inport  PortDimensions=20  SampleTime=0.01
      mask Display: e = 0.06;c1 = [120 230 180]/255;c2 = ([120 230 180]+0)/(256+128);c3 = ([120 230 180]+128)/(256+128);patch([0 1 1 0],[0 0 1 1],c1);patch([0 1 1 1-e 1-e 0+e],[0 0 1 1-e 0+e 0+e],c2);patch([0 0 1 1-e 0+e 0+e],[0 1 1 1-e 1-e 0+e],c3);plot([0 1 1 0 0],[0 0 1 1 0]);
  mux : Mux  Inputs=1
      mask Display: e = 0.06;c1 = [120 150 230]/255;c2 = ([120 150 230]+0)/383;c3 = ([120 150 230]+128)/383;patch([0 1 1 0],[0 0 1 1],c1);patch([0 1 1 1-e 1-e 0+e],[0 0 1 1-e 0+e 0+e],c2);patch([0 0 1 1-e 0+e 0+e],[0 1 1 1-e 1-e 0+e],c3);plot([0 1 1 0 0],[0 0 1 1 0]);disp('Mux')
  "pd{2,1}" : Outport
      mask Display: e = 0.06;c1 = [120 230 180]/255;c2 = ([120 230 180]+0)/(256+128);c3 = ([120 230 180]+128)/(256+128);patch([0 1 1 0],[0 0 1 1],c1);patch([0 1 1 1-e 1-e 0+e],[0 0 1 1-e 0+e 0+e],c2);patch([0 0 1 1-e 0+e 0+e],[0 1 1 1-e 1-e 0+e],c3);plot([0 1 1 0 0],[0 0 1 1 0]);
  wires:
  mux/1 -> "pd{2,1}"/1
  "p{2}"/1 -> mux/1

== system plant_n/PI Neural Network1/Layer 2/LW{2,1} ==
  "ad{2,1}" : Inport  PortDimensions=20  SampleTime=0.01
      mask Display: e = 0.06;c1 = [120 230 180]/255;c2 = ([120 230 180]+0)/(256+128);c3 = ([120 230 180]+128)/(256+128);patch([0 1 1 0],[0 0 1 1],c1);patch([0 1 1 1-e 1-e 0+e],[0 0 1 1-e 0+e 0+e],c2);patch([0 0 1 1-e 0+e 0+e],[0 1 1 1-e 1-e 0+e],c3);plot([0 1 1 0 0],[0 0 1 1 0]);
  "IW{2,1}(1,:)'" : Constant  Value=[0.045556080119317728105432507845762302167713642120361328125;-0.362754757442117992116692448689718730747699737548828125;-0.1903632995528562743547951185973943211138248443603515625;0.421154202195522187057719065705896355211734771728515625;0.2457853603451604918017636691729421727359294891357421875;0.303748793042679154918772610471933148801326751708984375;0.69307341668505595411176045672618784010410308837890625;-0.160688225653182137353525149592314846813678741455078125;0.5192167273493162316100324460421688854694366455078125;0.355402189105710586414232921015354804694652557373046875;0.376842823045455244113099979585967957973480224609375;0.005996473968998327318258301232845042250119149684906005859375;0.10049985067003076866232191832750686444342136383056640625;0.1562417704234825566178557210150756873190402984619140625;-0.12374642664488899601593629995477385818958282470703125;-0.462752702170863561281777265321579761803150177001953125;0.0602427026862962511355448214089847169816493988037109375;-0.31599478806734015989832187187857925891876220703125;0.2032721161179165125787449142080731689929962158203125;-0.46175958881991530091681852354668080806732177734375]
      mask Display: e = 0.06;c1 = [120 150 230]/255;c2 = ([120 150 230]+0)/383;c3 = ([120 150 230]+128)/383;patch([0 1 1 0],[0 0 1 1],c1);patch([0 1 1 1-e 1-e 0+e],[0 0 1 1-e 0+e 0+e],c2);patch([0 0 1 1-e 0+e 0+e],[0 1 1 1-e 1-e 0+e],c3);plot([0 1 1 0 0],[0 0 1 1 0]);disp('weights');
  Mux : Mux  Inputs=1
      mask Display: e = 0.06;c1 = [120 150 230]/255;c2 = ([120 150 230]+0)/383;c3 = ([120 150 230]+128)/383;patch([0 1 1 0],[0 0 1 1],c1);patch([0 1 1 1-e 1-e 0+e],[0 0 1 1-e 0+e 0+e],c2);patch([0 0 1 1-e 0+e 0+e],[0 1 1 1-e 1-e 0+e],c3);plot([0 1 1 0 0],[0 0 1 1 0]);disp('Mux');
  dotprod1 : neural/Weight Functions/dotprod
  "lz{2,1}" : Outport
      mask Display: e = 0.06;c1 = [120 230 180]/255;c2 = ([120 230 180]+0)/(256+128);c3 = ([120 230 180]+128)/(256+128);patch([0 1 1 0],[0 0 1 1],c1);patch([0 1 1 1-e 1-e 0+e],[0 0 1 1-e 0+e 0+e],c2);patch([0 0 1 1-e 0+e 0+e],[0 1 1 1-e 1-e 0+e],c3);plot([0 1 1 0 0],[0 0 1 1 0]);
  wires:
  Mux/1 -> "lz{2,1}"/1
  dotprod1/1 -> Mux/1
  "ad{2,1}"/1 -> dotprod1/2
  "IW{2,1}(1,:)'"/1 -> dotprod1/1
